simulink model "brakeSim"  (R2025a)
settings: Solver=VariableStepAuto  StartTime=0.0  StopTime=5  RelTol=1e-3
InitFcn:
  | init_params();
settings Model: Creator=PC5  LastModifiedBy=PC5

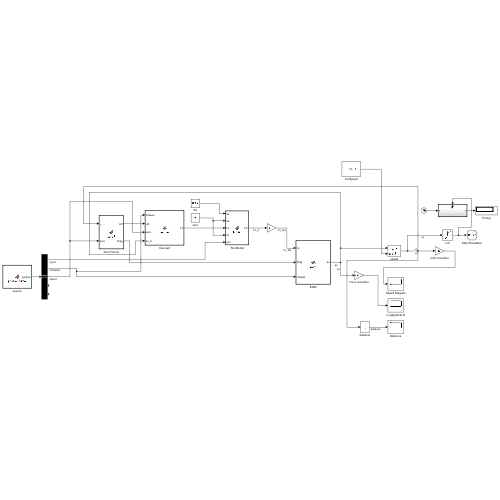
[thumbnail: Simulink's stored preview of the top-level diagram]
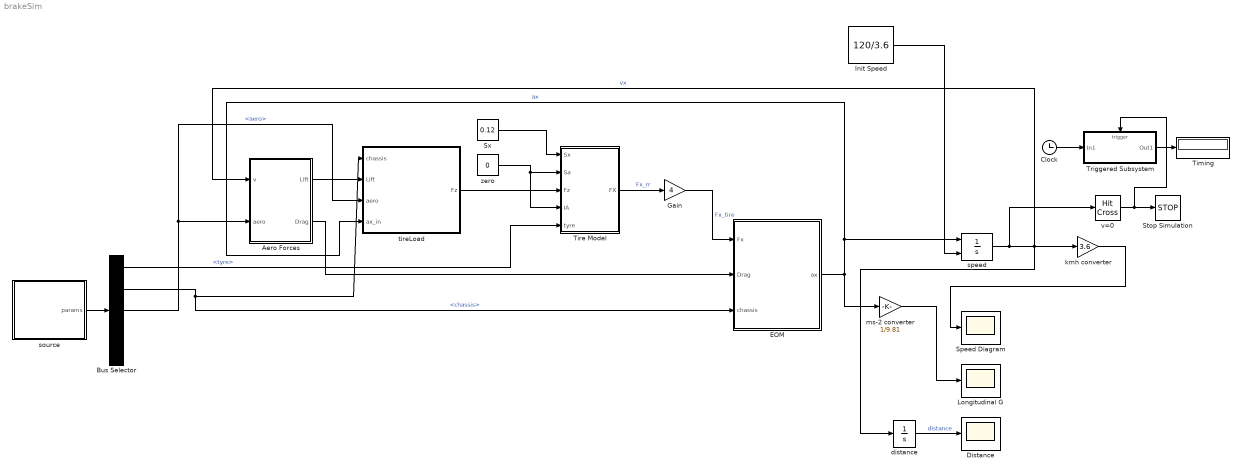
== system brakeSim ==
  Aero Forces : MATLAB Function  TreatAsAtomicUnit=on
  Bus Selector : BusSelector  OutputSignals=tyre,chassis,aero,pwt,suspension
  Clock : Clock
  Distance : Scope
      settings: ActiveDisplayYMinimum=-11.396111735556595  ActiveDisplayYMaximum=85.165070742986842
  EOM : MATLAB Function  TreatAsAtomicUnit=on
  Gain : Gain  Gain=4
  Init Speed : Constant  Value=120/3.6
  Longitudinal G : Scope
      settings: ActiveDisplayYMinimum=-1  ActiveDisplayYMaximum=1  DataLoggingVariableName=ScopeData2
  Speed Diagram : Scope
      settings: ActiveDisplayYMinimum=-14.999999999999998  ActiveDisplayYMaximum=135.00000000000003
  Stop Simulation : Stop
  Sx : Constant  Value=0.12
  Timing : Display
  Tire Model : MATLAB Function  TreatAsAtomicUnit=on
  Triggered Subsystem : Subsystem  TreatAsAtomicUnit=on
  distance : Integrator
  kmh converter : Gain  Gain=3.6
  ms-2 converter : Gain  Gain=1/9.81
  source : MATLAB Function  TreatAsAtomicUnit=on
  speed : Integrator  InitialConditionSource=external  LimitOutput=on  LowerSaturationLimit=0
  tireLoad : MATLAB Function  TreatAsAtomicUnit=on
  v=0 : HitCross  HitCrossingOffset=0.001  HitCrossingDirection=rising
  zero : Constant  Value=0
  wires:
  Aero Forces/1(Lift) -> tireLoad/2(Lift)
  Aero Forces/2(Drag) -> EOM/2(Drag)
  EOM/1(ax) -> ms-2 converter/1, speed/1, tireLoad/4(ax_in)  "ax"
  speed/1 -> distance/1, kmh converter/1, Aero Forces/1(v), v=0/1  "vx"
  Tire Model/1(FX) -> Gain/1  "Fx_rr"
  zero/1 -> Tire Model/4(IA), Tire Model/2(Sa)
  tireLoad/1(Fz) -> Tire Model/3(Fz)
  Sx/1 -> Tire Model/1(Sx)
  source/1(params) -> Bus Selector/1
  Bus Selector/1 -> Tire Model/5(tyre)  "<tyre>"
  Bus Selector/2 -> EOM/3(chassis), tireLoad/1(chassis)  "<chassis>"
  Bus Selector/3 -> Aero Forces/2(aero), tireLoad/3(aero)  "<aero>"
  kmh converter/1 -> Speed Diagram/1
  ms-2 converter/1 -> Longitudinal G/1
  Init Speed/1 -> speed/2
  v=0/1 -> Triggered Subsystem/Trigger, Stop Simulation/1
  distance/1 -> Distance/1  "distance"
  Gain/1 -> EOM/1(Fx)  "Fx_tire"
  Clock/1 -> Triggered Subsystem/1(In1)
  Triggered Subsystem/1(Out1) -> Timing/1

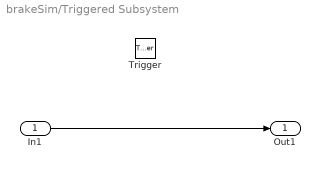
== system brakeSim/Triggered Subsystem ==
  In1 : Inport
  Trigger : TriggerPort  VariantControl=(inherit)
  Out1 : Outport
  wires:
  In1/1 -> Out1/1

== matlab function brakeSim/Tire Model ==
  data: FX output; Sx input; Sa input; Fz input; IA input; tyre input
function FX = MF52(Sx, Sa, Fz, IA, tyre)
%#codegen
% MF5.2 Combined-slip Longitudinal Force (FX)
% Inputs:  Sx (kappa), Sa (alpha, deg), Fz (N), IA (deg)
% Uses workspace tyre struct: tyre.<field> (plain doubles)

%% Constants
cf = 0.55;   % grip factor

%% Nominal load
FZ0 = tyre.FZ0;

KAPPA = Sx;          % [-]
ALPHA = Sa;          % [deg]
FZ    = Fz;          % [N]
GAMMA = IA*pi/180;   % [rad]

LFZO  = tyre.LFZO;
FZ0PR = FZ0 * LFZO;
DFZ   = (FZ - FZ0PR) ./ FZ0PR;

%% Scaling Factors
LGAY = tyre.LGAY;
LHY  = tyre.LHY;
LVY  = tyre.LVY;
LCY  = tyre.LCY;
LEY  = tyre.LEY;
LHX  = tyre.LHX;
LVX  = tyre.LVX;
LGX  = tyre.LGX;
LCX  = tyre.LCX;
LEX  = tyre.LEX;
LXAL = tyre.LXAL;

LKY  = tyre.LKY;
LKX  = tyre.LKX;
LMUY = cf * tyre.LMUY;
LMUX = cf * tyre.LMUX;

%% Longitudinal Coefficients
PCX1 = tyre.PCX1;
PDX1 = tyre.PDX1;
PDX2 = tyre.PDX2;
PDX3 = tyre.PDX3;
PEX1 = tyre.PEX1;
PEX2 = tyre.PEX2;
PEX3 = tyre.PEX3;
PEX4 = tyre.PEX4;
PKX1 = tyre.PKX1;
PKX2 = tyre.PKX2;
PKX3 = tyre.PKX3;
PHX1 = tyre.PHX1;
PHX2 = tyre.PHX2;
PVX1 = tyre.PVX1;
PVX2 = tyre.PVX2;

%% Combined Longitudinal Coefficients
RBX1 = tyre.RBX1;
RBX2 = tyre.RBX2;
RCX1 = tyre.RCX1;
REX1 = tyre.REX1;
REX2 = tyre.REX2;
RHX1 = tyre.RHX1;

%% Lateral Coefficients (needed for combined slip)
PCY1 = tyre.PCY1;
PDY1 = tyre.PDY1;
PDY2 = tyre.PDY2;
PDY3 = tyre.PDY3;
PEY1 = tyre.PEY1;
PEY2 = tyre.PEY2;
PEY3 = tyre.PEY3;
PEY4 = tyre.PEY4;
PKY1 = tyre.PKY1;
PKY2 = tyre.PKY2;
PKY3 = tyre.PKY3;
PHY1 = tyre.PHY1;
PHY2 = tyre.PHY2;
PHY3 = tyre.PHY3;
PVY1 = tyre.PVY1;
PVY2 = tyre.PVY2;
PVY3 = tyre.PVY3;
PVY4 = tyre.PVY4;

%% Combined Lateral Coefficients
RBY1 = tyre.RBY1;
RBY2 = tyre.RBY2;
RBY3 = tyre.RBY3;
RCY1 = tyre.RCY1;
REY1 = tyre.REY1;
REY2 = tyre.REY2;
RHY1 = tyre.RHY1;
RHY2 = tyre.RHY2;
RVY1 = tyre.RVY1;
RVY2 = tyre.RVY2;
RVY3 = tyre.RVY3;
RVY4 = tyre.RVY4;
RVY5 = tyre.RVY5;
RVY6 = tyre.RVY6;

%% ---------- Lateral Force FY (for combined-slip factors) ----------
GAMMAY = GAMMA .* LGAY;
SHY    = (PHY1 + PHY2.*DFZ).*LHY + PHY3.*GAMMAY;

SVY    = 0;
ALPHAY = ALPHA + SHY;

CY  = PCY1 .* LCY;
MUY = (PDY1 + PDY2.*DFZ) .* (1 - PDY3.*(GAMMAY.^2)) .* LMUY;
DY  = MUY .* FZ;
EY  = (PEY1 + PEY2.*DFZ) .* ...
      (1 - (PEY3 + PEY4.*GAMMAY).*sign(ALPHAY)) .* LEY;

KY0 = PKY1 .* FZ0 .* sin(2.*atan(FZ./(PKY2.*FZ0PR))) .* LKY;
KY  = KY0 .* (1 - PKY3.*abs(GAMMAY));
BY  = KY ./ (CY.*DY);

FY0 = DY .* sin(CY.*atan(BY.*ALPHAY - EY.*(BY.*ALPHAY - atan(BY.*ALPHAY)))) + SVY;

BYK  = RBY1 .* cos(atan(RBY2.*(ALPHA - RBY3)));
CYK  = RCY1;
EYK  = REY1 + REY2.*DFZ;
SHYK = RHY1 + RHY2.*DFZ;

KS   = KAPPA + SHYK;
DVYK = MUY.*FZ .* (RVY1 + RVY2.*DFZ + RVY3.*GAMMA) .* cos(atan(RVY4.*ALPHA));
SVYK = DVYK .* sin(RVY5.*atan(RVY6.*KAPPA));

DYK = FY0 ./ ...
      (cos(CYK.*atan(BYK.*SHYK - EYK.*(BYK.*SHYK - atan(BYK.*SHYK)))));

GYK = (cos(CYK.*atan(BYK.*KS - EYK.*(BYK.*KS - atan(BYK.*KS))))) ./ ...
      (cos(CYK.*atan(BYK.*SHYK - EYK.*(BYK.*SHYK - atan(BYK.*SHYK)))));

FY = GYK.*FY0 + SVYK; %#ok<NASGU>

%% ---------- Longitudinal Force FX ----------
SHX = (PHX1 + PHX2.*DFZ).*LHX;
SVX = FZ .* (PVX1 + PVX2.*DFZ) .* LVX .* LMUX;

KAPPAX = KAPPA + SHX;
GAMMAX = GAMMA .* LGX; %#ok<NASGU>

CX  = PCX1 .* LCX;
MUX = (PDX1 + PDX2.*DFZ) .* (1 - PDX3.*(GAMMA.^2)) .* LMUX;
DX  = MUX .* FZ;

EX = (PEX1 + PEX2.*DFZ + PEX3.*(DFZ.^2)) .* ...
     (1 - PEX4.*sign(KAPPAX)) .* LEX;

KX = FZ .* (PKX1 + PKX2.*DFZ) .* exp(PKX3.*DFZ) .* LKX;
BX = KX ./ (CX.*DX);

FX0 = DX .* sin(CX.*atan(BX.*KAPPAX - EX.*(BX.*KAPPAX - atan(BX.*KAPPAX))) + SVX);

SHXAL  = RHX1;
CXAL   = RCX1;
BXAL   = RBX1 .* cos(atan(RBX2.*KAPPA)) .* LXAL;
ALPHAS = ALPHA + SHXAL;
EXAL   = REX1 + REX2.*DFZ;

GXAL = (cos(CXAL.*atan(BXAL.*ALPHAS - EXAL.*(BXAL.*ALPHAS - atan(BXAL.*ALPHAS))))) ./ ...
       (cos(CXAL.*atan(BXAL.*SHXAL  - EXAL.*(BXAL.*SHXAL  - atan(BXAL.*SHXAL )))));

FX = GXAL .* FX0;
end

== matlab function brakeSim/Aero Forces ==
  data: Lift output; Drag output; v input; aero input
% calculates aerodynamics

function [Lift, Drag] = aeroF(v,aero)

Lift = 0.5*aero.farea*aero.CLs*aero.den*v^2;
Drag = 0.5*aero.farea*aero.CDs*aero.den*v^2;


end

== matlab function brakeSim/tireLoad ==
  data: chassis input; Lift input; Fz output; aero input; ax_in input
function Fz = tireLoad(chassis,Lift,aero,ax_in)

mass = chassis.car+chassis.driver;
ab = aero.ab_s;
cg_h = chassis.cg_h;
wheelbase = chassis.wheelbase;

% normal load by mass
Fz = (mass*9.81)/4;
% aero downforce
AeroR = Lift*(1-ab);
% load transfer
longLT = Fz*(ax_in/9.81)*cg_h/wheelbase;
% wheel loads per wheel
Fz= Fz+AeroR/2+longLT/2;

end

== matlab function brakeSim/EOM ==
  data: Fx input; ax output; Drag input; chassis input
function ax  = EOM(Fx,Drag,chassis)
ax = (Fx-Drag)/(chassis.driver+chassis.car);
end

== matlab function brakeSim/source ==
  data: params output Bus: ParamsBus; PARAMS parameter Bus: ParamsBus
function params = paramSource(PARAMS)
%#codegen
params = PARAMS;
end
